simulink model "Dynamics"  (R2023a)
settings: Solver=FixedStepAuto  StartTime=0.0  StopTime=inf  FixedStep=0.001  EnableMultiTasking=on
libraries: sharedutil x32, sharedtransform x18, dspmtrx3 x12, matrix_library x6, simulink_extras x1, simulink x1
(part 3 of 6)

== system Dynamics/Subsystem/M(q),C(q,dq),g(q)/G gen ==
  m : Inport
  Demux : Demux  Outputs=6
  Mux : Mux  Inputs=7
  Product{,1..5} (6 alike) : Product
  g : Constant  Value=[0;0;9.81]
  g1 : Constant  Value=zeros(18,1)
  G : Outport
  wires:
  m/1 -> Demux/1
  Demux/1 -> Product/1
  Demux/2 -> Product1/1
  Demux/3 -> Product2/1
  g/1 -> Product5/2, Product4/2, Product3/2, Product2/2, Product1/2, Product/2
  Demux/4 -> Product3/1
  Demux/5 -> Product4/1
  Demux/6 -> Product5/1
  Product1/1 -> Mux/2
  Product/1 -> Mux/1
  Product2/1 -> Mux/3
  Product4/1 -> Mux/5
  Product5/1 -> Mux/6
  Product3/1 -> Mux/4
  g1/1 -> Mux/7
  Mux/1 -> G/1

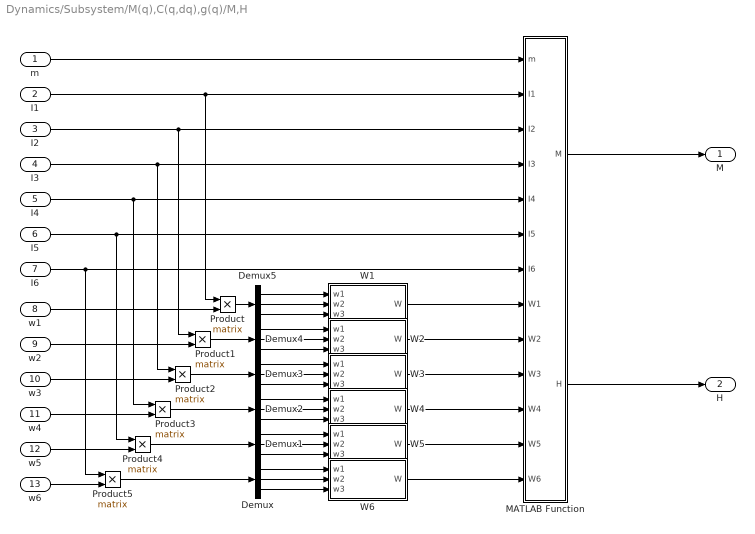
== system Dynamics/Subsystem/M(q),C(q,dq),g(q)/M,H ==
  m : Inport
  I1 : Inport  Port=2
  I2 : Inport  Port=3
  I3 : Inport  Port=4
  I4 : Inport  Port=5
  I5 : Inport  Port=6
  I6 : Inport  Port=7
  w1 : Inport  Port=8
  w2 : Inport  Port=9
  w3 : Inport  Port=10
  w4 : Inport  Port=11
  w5 : Inport  Port=12
  w6 : Inport  Port=13
  Demux{,1..5} (6 alike) : Demux  Outputs=3
  MATLAB Function : MATLAB Function  TreatAsAtomicUnit=on
  Product{,1..5} (6 alike) : Product  Multiplication=Matrix(*)
  W1 : MATLAB Function  TreatAsAtomicUnit=on
  W2 : MATLAB Function  TreatAsAtomicUnit=on
  W3 : MATLAB Function  TreatAsAtomicUnit=on
  W4 : MATLAB Function  TreatAsAtomicUnit=on
  W5 : MATLAB Function  TreatAsAtomicUnit=on
  W6 : MATLAB Function  TreatAsAtomicUnit=on
  M : Outport
  H : Outport  Port=2
  wires:
  m/1 -> MATLAB Function/1(m)
  I1/1 -> Product/1, MATLAB Function/2(I1)
  I2/1 -> Product1/1, MATLAB Function/3(I2)
  I3/1 -> Product2/1, MATLAB Function/4(I3)
  I4/1 -> Product3/1, MATLAB Function/5(I4)
  I5/1 -> Product4/1, MATLAB Function/6(I5)
  I6/1 -> Product5/1, MATLAB Function/7(I6)
  MATLAB Function/1(M) -> M/1
  MATLAB Function/2(H) -> H/1
  W1/1(W) -> MATLAB Function/8(W1)
  W2/1(W) -> MATLAB Function/9(W2)
  W3/1(W) -> MATLAB Function/10(W3)
  W4/1(W) -> MATLAB Function/11(W4)
  W5/1(W) -> MATLAB Function/12(W5)
  W6/1(W) -> MATLAB Function/13(W6)
  w6/1 -> Product5/2
  Demux/3 -> W6/3(w3)
  Demux/2 -> W6/2(w2)
  Demux/1 -> W6/1(w1)
  w5/1 -> Product4/2
  Demux1/3 -> W5/3(w3)
  Demux1/2 -> W5/2(w2)
  Demux1/1 -> W5/1(w1)
  w4/1 -> Product3/2
  Demux2/3 -> W4/3(w3)
  Demux2/2 -> W4/2(w2)
  Demux2/1 -> W4/1(w1)
  w3/1 -> Product2/2
  Demux3/3 -> W3/3(w3)
  Demux3/2 -> W3/2(w2)
  Demux3/1 -> W3/1(w1)
  w2/1 -> Product1/2
  Demux4/3 -> W2/3(w3)
  Demux4/2 -> W2/2(w2)
  Demux4/1 -> W2/1(w1)
  w1/1 -> Product/2
  Demux5/3 -> W1/3(w3)
  Demux5/2 -> W1/2(w2)
  Demux5/1 -> W1/1(w1)
  Product/1 -> Demux5/1
  Product1/1 -> Demux4/1
  Product2/1 -> Demux3/1
  Product3/1 -> Demux2/1
  Product4/1 -> Demux1/1
  Product5/1 -> Demux/1

== system Dynamics/Subsystem/Moments of inertia/Ix, Iy ==
  r : Inport
  m : Inport  Port=2
  h : Inport  Port=3
  Add : Sum
  Gain : Gain  Gain=3
  Gain1 : Gain  Gain=1/12
  Product : Product
  Product1 : Product
  Product2 : Product
  Iz : Outport
  wires:
  r/1 -> Product/1, Product/2
  h/1 -> Product1/1, Product1/2
  Product/1 -> Gain/1
  Product1/1 -> Add/2
  Add/1 -> Product2/1
  m/1 -> Product2/2
  Gain/1 -> Add/1
  Product2/1 -> Gain1/1
  Gain1/1 -> Iz/1

== system Dynamics/Subsystem/Moments of inertia/Ix, Iy1 ==
  r : Inport
  m : Inport  Port=2
  h : Inport  Port=3
  Add : Sum
  Gain : Gain  Gain=3
  Gain1 : Gain  Gain=1/12
  Product : Product
  Product1 : Product
  Product2 : Product
  Iz : Outport
  wires:
  r/1 -> Product/1, Product/2
  h/1 -> Product1/1, Product1/2
  Product/1 -> Gain/1
  Product1/1 -> Add/2
  Add/1 -> Product2/1
  m/1 -> Product2/2
  Gain/1 -> Add/1
  Product2/1 -> Gain1/1
  Gain1/1 -> Iz/1

== system Dynamics/Subsystem/Moments of inertia/Ix, Iy2 ==
  r : Inport
  m : Inport  Port=2
  h : Inport  Port=3
  Add : Sum
  Gain : Gain  Gain=3
  Gain1 : Gain  Gain=1/12
  Product : Product
  Product1 : Product
  Product2 : Product
  Iz : Outport
  wires:
  r/1 -> Product/1, Product/2
  h/1 -> Product1/1, Product1/2
  Product/1 -> Gain/1
  Product1/1 -> Add/2
  Add/1 -> Product2/1
  m/1 -> Product2/2
  Gain/1 -> Add/1
  Product2/1 -> Gain1/1
  Gain1/1 -> Iz/1

== system Dynamics/Subsystem/Moments of inertia/Ix, Iy3 ==
  r : Inport
  m : Inport  Port=2
  h : Inport  Port=3
  Add : Sum
  Gain : Gain  Gain=3
  Gain1 : Gain  Gain=1/12
  Product : Product
  Product1 : Product
  Product2 : Product
  Iz : Outport
  wires:
  r/1 -> Product/1, Product/2
  h/1 -> Product1/1, Product1/2
  Product/1 -> Gain/1
  Product1/1 -> Add/2
  Add/1 -> Product2/1
  m/1 -> Product2/2
  Gain/1 -> Add/1
  Product2/1 -> Gain1/1
  Gain1/1 -> Iz/1

== system Dynamics/Subsystem/Moments of inertia/Ix, Iy4 ==
  r : Inport
  m : Inport  Port=2
  h : Inport  Port=3
  Add : Sum
  Gain : Gain  Gain=3
  Gain1 : Gain  Gain=1/12
  Product : Product
  Product1 : Product
  Product2 : Product
  Iz : Outport
  wires:
  r/1 -> Product/1, Product/2
  h/1 -> Product1/1, Product1/2
  Product/1 -> Gain/1
  Product1/1 -> Add/2
  Add/1 -> Product2/1
  m/1 -> Product2/2
  Gain/1 -> Add/1
  Product2/1 -> Gain1/1
  Gain1/1 -> Iz/1

== system Dynamics/Subsystem/Moments of inertia/Ix, Iy5 ==
  r : Inport
  m : Inport  Port=2
  h : Inport  Port=3
  Add : Sum
  Gain : Gain  Gain=3
  Gain1 : Gain  Gain=1/12
  Product : Product
  Product1 : Product
  Product2 : Product
  Iz : Outport
  wires:
  r/1 -> Product/1, Product/2
  h/1 -> Product1/1, Product1/2
  Product/1 -> Gain/1
  Product1/1 -> Add/2
  Add/1 -> Product2/1
  m/1 -> Product2/2
  Gain/1 -> Add/1
  Product2/1 -> Gain1/1
  Gain1/1 -> Iz/1

== system Dynamics/Subsystem/Moments of inertia/Iz ==
  r : Inport
  m : Inport  Port=2
  Constant : Constant  Value=0.5
  Product : Product  Inputs=4
  Iz : Outport
  wires:
  m/1 -> Product/3
  Constant/1 -> Product/4
  r/1 -> Product/2, Product/1
  Product/1 -> Iz/1

== system Dynamics/Subsystem/Moments of inertia/Iz1 ==
  r : Inport
  m : Inport  Port=2
  Constant : Constant  Value=0.5
  Product : Product  Inputs=4
  Iz : Outport
  wires:
  m/1 -> Product/3
  Constant/1 -> Product/4
  r/1 -> Product/2, Product/1
  Product/1 -> Iz/1

== system Dynamics/Subsystem/Moments of inertia/Iz2 ==
  r : Inport
  m : Inport  Port=2
  Constant : Constant  Value=0.5
  Product : Product  Inputs=4
  Iz : Outport
  wires:
  m/1 -> Product/3
  Constant/1 -> Product/4
  r/1 -> Product/2, Product/1
  Product/1 -> Iz/1

== system Dynamics/Subsystem/Moments of inertia/Iz3 ==
  r : Inport
  m : Inport  Port=2
  Constant : Constant  Value=0.5
  Product : Product  Inputs=4
  Iz : Outport
  wires:
  m/1 -> Product/3
  Constant/1 -> Product/4
  r/1 -> Product/2, Product/1
  Product/1 -> Iz/1

== system Dynamics/Subsystem/Moments of inertia/Iz4 ==
  r : Inport
  m : Inport  Port=2
  Constant : Constant  Value=0.5
  Product : Product  Inputs=4
  Iz : Outport
  wires:
  m/1 -> Product/3
  Constant/1 -> Product/4
  r/1 -> Product/2, Product/1
  Product/1 -> Iz/1

== system Dynamics/Subsystem/Moments of inertia/Iz5 ==
  r : Inport
  m : Inport  Port=2
  Constant : Constant  Value=0.5
  Product : Product  Inputs=4
  Iz : Outport
  wires:
  m/1 -> Product/3
  Constant/1 -> Product/4
  r/1 -> Product/2, Product/1
  Product/1 -> Iz/1

== system Dynamics/Subsystem/Slotine/S-gen ==
  dq : Inport
  V : Inport  Port=2
  Gain : Gain  Gain=-1
  Sum : Sum  Inputs=|++
  S : Outport
  wires:
  dq/1 -> Sum/1
  Sum/1 -> S/1
  V/1 -> Gain/1
  Gain/1 -> Sum/2

== system Dynamics/Subsystem/Slotine/V-gen ==
  q_tilde : Inport
  dq_d : Inport  Port=2
  Gamma : Inport  Port=3
  Gain : Gain  Gain=-1
  Product : Product  Multiplication=Matrix(*)
  Sum : Sum  Inputs=|++
  V : Outport
  wires:
  Gamma/1 -> Product/1
  q_tilde/1 -> Product/2
  Product/1 -> Gain/1
  Sum/1 -> V/1
  dq_d/1 -> Sum/1
  Gain/1 -> Sum/2

== system Dynamics/Subsystem/Slotine/dV-gen ==
  dq_tilde : Inport
  ddq_d : Inport  Port=2
  Gamma : Inport  Port=3
  Gain : Gain  Gain=-1
  Product : Product  Multiplication=Matrix(*)
  Sum : Sum  Inputs=|++
  dV : Outport
  wires:
  Gamma/1 -> Product/1
  dq_tilde/1 -> Product/2
  Product/1 -> Gain/1
  Sum/1 -> dV/1
  ddq_d/1 -> Sum/1
  Gain/1 -> Sum/2

== system Dynamics/Subsystem/Slotine/tau-gen ==
  M : Inport
  C : Inport  Port=2
  g : Inport  Port=3
  V : Inport  Port=4
  dV : Inport  Port=5
  S : Inport  Port=6
  K : Inport  Port=7
  u0 : Inport  Port=8
  Product : Product  Multiplication=Matrix(*)
  Product1 : Product  Multiplication=Matrix(*)
  Product2 : Product  Multiplication=Matrix(*)
  Sum : Sum  Inputs=|++
  Sum1 : Sum  Inputs=|++
  Sum2 : Sum  Inputs=|+-
  Sum3 : Sum  Inputs=|++
  tau : Outport
  wires:
  M/1 -> Product/1
  dV/1 -> Product/2
  C/1 -> Product1/1
  V/1 -> Product1/2
  S/1 -> Product2/2
  K/1 -> Product2/1
  Product/1 -> Sum/1
  Product1/1 -> Sum/2
  Sum/1 -> Sum1/1
  g/1 -> Sum1/2
  Product2/1 -> Sum2/2
  Sum1/1 -> Sum2/1
  Sum2/1 -> Sum3/1
  Sum3/1 -> tau/1
  u0/1 -> Sum3/2

== system Dynamics/Subsystem/Slotine/u0-gen ==
  S : Inport
  sigma(t) : Inport  Port=2
  Divide : Product  Inputs=*/
  Dot Product : DotProduct  OutDataTypeStr=Inherit: Inherit via internal rule
  Gain : Gain  Gain=-1
  Product : Product
  Product1 : Product
  Product2 : Product
  Sqrt : Sqrt
  Sum : Sum  Inputs=|++
  gamma_hat : Integrator  InitialCondition=1
  u0 : Outport
  wires:
  gamma_hat/1 -> Product2/1, Product/2, Product/1
  Dot Product/1 -> Sqrt/1
  S/1 -> Product1/2, Dot Product/2, Dot Product/1
  Sqrt/1 -> Product2/2, gamma_hat/1
  Product/1 -> Product1/1
  Product1/1 -> Divide/1
  Product2/1 -> Sum/1
  Sum/1 -> Divide/2
  sigma(t)/1 -> Sum/2
  Divide/1 -> Gain/1
  Gain/1 -> u0/1

== system Dynamics/Subsystem2/H_6^0/H_1^0 ==
  a : Inport
  alpha : Inport  Port=2
  theta : Inport  Port=3
  d : Inport  Port=4
  Gain1 : Gain  Gain=-1
  Gain2 : Gain  Gain=-1
  MATLAB Function : MATLAB Function  TreatAsAtomicUnit=on
  Mux : Mux  Inputs=3
  Mux1 : Mux  Inputs=3
  Product : Product
  Product1 : Product
  Rotation Angles to Direction Cosine Matrix : sharedtransform/Rotation Angles to Direction Cosine Matrix  rotationOrder=ZXY  aMode=aMode
  Trigonometric Function : Trigonometry  Operator=cos
  Trigonometric Function1 : Trigonometry
  Zero : Constant  Value=0
  H : Outport
  R : Outport  Port=2
  p : Outport  Port=3
  wires:
  Mux/1 -> Rotation Angles to Direction Cosine Matrix/1
  alpha/1 -> Gain1/1
  Zero/1 -> Mux/3
  Rotation Angles to Direction Cosine Matrix/1 -> MATLAB Function/1(R), R/1
  Mux1/1 -> MATLAB Function/2(p), p/1
  Trigonometric Function/1 -> Product/1
  Trigonometric Function1/1 -> Product1/1
  Product/1 -> Mux1/1
  Product1/1 -> Mux1/2
  a/1 -> Product/2, Product1/2
  MATLAB Function/1(H) -> H/1
  Gain1/1 -> Mux/1
  Gain2/1 -> Mux/2
  theta/1 -> Trigonometric Function1/1, Trigonometric Function/1, Gain2/1
  d/1 -> Mux1/3

== system Dynamics/Subsystem2/H_6^0/H_2^1 ==
  a : Inport
  alpha : Inport  Port=2
  theta : Inport  Port=3
  d : Inport  Port=4
  Gain1 : Gain  Gain=-1
  Gain2 : Gain  Gain=-1
  MATLAB Function : MATLAB Function  TreatAsAtomicUnit=on
  Mux : Mux  Inputs=3
  Mux1 : Mux  Inputs=3
  Product : Product
  Product1 : Product
  Rotation Angles to Direction Cosine Matrix : sharedtransform/Rotation Angles to Direction Cosine Matrix  rotationOrder=ZXY  aMode=aMode
  Trigonometric Function : Trigonometry  Operator=cos
  Trigonometric Function1 : Trigonometry
  Zero : Constant  Value=0
  H : Outport
  R : Outport  Port=2
  p : Outport  Port=3
  wires:
  Mux/1 -> Rotation Angles to Direction Cosine Matrix/1
  alpha/1 -> Gain1/1
  Zero/1 -> Mux/3
  Rotation Angles to Direction Cosine Matrix/1 -> MATLAB Function/1(R), R/1
  Mux1/1 -> MATLAB Function/2(p), p/1
  Trigonometric Function/1 -> Product/1
  Trigonometric Function1/1 -> Product1/1
  Product/1 -> Mux1/1
  Product1/1 -> Mux1/2
  a/1 -> Product/2, Product1/2
  MATLAB Function/1(H) -> H/1
  Gain1/1 -> Mux/1
  Gain2/1 -> Mux/2
  theta/1 -> Trigonometric Function1/1, Trigonometric Function/1, Gain2/1
  d/1 -> Mux1/3

== system Dynamics/Subsystem2/H_6^0/H_3^2 ==
  a : Inport
  alpha : Inport  Port=2
  theta : Inport  Port=3
  d : Inport  Port=4
  Gain1 : Gain  Gain=-1
  Gain2 : Gain  Gain=-1
  MATLAB Function : MATLAB Function  TreatAsAtomicUnit=on
  Mux : Mux  Inputs=3
  Mux1 : Mux  Inputs=3
  Product : Product
  Product1 : Product
  Rotation Angles to Direction Cosine Matrix : sharedtransform/Rotation Angles to Direction Cosine Matrix  rotationOrder=ZXY  aMode=aMode
  Trigonometric Function : Trigonometry  Operator=cos
  Trigonometric Function1 : Trigonometry
  Zero : Constant  Value=0
  H : Outport
  R : Outport  Port=2
  p : Outport  Port=3
  wires:
  Mux/1 -> Rotation Angles to Direction Cosine Matrix/1
  alpha/1 -> Gain1/1
  Zero/1 -> Mux/3
  Rotation Angles to Direction Cosine Matrix/1 -> MATLAB Function/1(R), R/1
  Mux1/1 -> MATLAB Function/2(p), p/1
  Trigonometric Function/1 -> Product/1
  Trigonometric Function1/1 -> Product1/1
  Product/1 -> Mux1/1
  Product1/1 -> Mux1/2
  a/1 -> Product/2, Product1/2
  MATLAB Function/1(H) -> H/1
  Gain1/1 -> Mux/1
  Gain2/1 -> Mux/2
  theta/1 -> Trigonometric Function1/1, Trigonometric Function/1, Gain2/1
  d/1 -> Mux1/3

== system Dynamics/Subsystem2/H_6^0/H_4^3 ==
  a : Inport
  alpha : Inport  Port=2
  theta : Inport  Port=3
  d : Inport  Port=4
  Gain1 : Gain  Gain=-1
  Gain2 : Gain  Gain=-1
  MATLAB Function : MATLAB Function  TreatAsAtomicUnit=on
  Mux : Mux  Inputs=3
  Mux1 : Mux  Inputs=3
  Product : Product
  Product1 : Product
  Rotation Angles to Direction Cosine Matrix : sharedtransform/Rotation Angles to Direction Cosine Matrix  rotationOrder=ZXY  aMode=aMode
  Trigonometric Function : Trigonometry  Operator=cos
  Trigonometric Function1 : Trigonometry
  Zero : Constant  Value=0
  H : Outport
  R : Outport  Port=2
  p : Outport  Port=3
  wires:
  Mux/1 -> Rotation Angles to Direction Cosine Matrix/1
  alpha/1 -> Gain1/1
  Zero/1 -> Mux/3
  Rotation Angles to Direction Cosine Matrix/1 -> MATLAB Function/1(R), R/1
  Mux1/1 -> MATLAB Function/2(p), p/1
  Trigonometric Function/1 -> Product/1
  Trigonometric Function1/1 -> Product1/1
  Product/1 -> Mux1/1
  Product1/1 -> Mux1/2
  a/1 -> Product/2, Product1/2
  MATLAB Function/1(H) -> H/1
  Gain1/1 -> Mux/1
  Gain2/1 -> Mux/2
  theta/1 -> Trigonometric Function1/1, Trigonometric Function/1, Gain2/1
  d/1 -> Mux1/3

== system Dynamics/Subsystem2/H_6^0/H_5^4 ==
  a : Inport
  alpha : Inport  Port=2
  theta : Inport  Port=3
  d : Inport  Port=4
  Gain1 : Gain  Gain=-1
  Gain2 : Gain  Gain=-1
  MATLAB Function : MATLAB Function  TreatAsAtomicUnit=on
  Mux : Mux  Inputs=3
  Mux1 : Mux  Inputs=3
  Product : Product
  Product1 : Product
  Rotation Angles to Direction Cosine Matrix : sharedtransform/Rotation Angles to Direction Cosine Matrix  rotationOrder=ZXY  aMode=aMode
  Trigonometric Function : Trigonometry  Operator=cos
  Trigonometric Function1 : Trigonometry
  Zero : Constant  Value=0
  H : Outport
  R : Outport  Port=2
  p : Outport  Port=3
  wires:
  Mux/1 -> Rotation Angles to Direction Cosine Matrix/1
  alpha/1 -> Gain1/1
  Zero/1 -> Mux/3
  Rotation Angles to Direction Cosine Matrix/1 -> MATLAB Function/1(R), R/1
  Mux1/1 -> MATLAB Function/2(p), p/1
  Trigonometric Function/1 -> Product/1
  Trigonometric Function1/1 -> Product1/1
  Product/1 -> Mux1/1
  Product1/1 -> Mux1/2
  a/1 -> Product/2, Product1/2
  MATLAB Function/1(H) -> H/1
  Gain1/1 -> Mux/1
  Gain2/1 -> Mux/2
  theta/1 -> Trigonometric Function1/1, Trigonometric Function/1, Gain2/1
  d/1 -> Mux1/3

== system Dynamics/Subsystem2/H_6^0/H_6^5 ==
  a : Inport
  alpha : Inport  Port=2
  theta : Inport  Port=3
  d : Inport  Port=4
  Gain1 : Gain  Gain=-1
  Gain2 : Gain  Gain=-1
  MATLAB Function : MATLAB Function  TreatAsAtomicUnit=on
  Mux : Mux  Inputs=3
  Mux1 : Mux  Inputs=3
  Product : Product
  Product1 : Product
  Rotation Angles to Direction Cosine Matrix : sharedtransform/Rotation Angles to Direction Cosine Matrix  rotationOrder=ZXY  aMode=aMode
  Trigonometric Function : Trigonometry  Operator=cos
  Trigonometric Function1 : Trigonometry
  Zero : Constant  Value=0
  H : Outport
  R : Outport  Port=2
  p : Outport  Port=3
  wires:
  Mux/1 -> Rotation Angles to Direction Cosine Matrix/1
  alpha/1 -> Gain1/1
  Zero/1 -> Mux/3
  Rotation Angles to Direction Cosine Matrix/1 -> MATLAB Function/1(R), R/1
  Mux1/1 -> MATLAB Function/2(p), p/1
  Trigonometric Function/1 -> Product/1
  Trigonometric Function1/1 -> Product1/1
  Product/1 -> Mux1/1
  Product1/1 -> Mux1/2
  a/1 -> Product/2, Product1/2
  MATLAB Function/1(H) -> H/1
  Gain1/1 -> Mux/1
  Gain2/1 -> Mux/2
  theta/1 -> Trigonometric Function1/1, Trigonometric Function/1, Gain2/1
  d/1 -> Mux1/3

== system Dynamics/Subsystem2/Jacobian/J(q) gen. ==
  R_1^0 : Inport
  R_2^0 : Inport  Port=2
  R_3^0 : Inport  Port=3
  R_4^0 : Inport  Port=4
  R_5^0 : Inport  Port=5
  R_6^0 : Inport  Port=6
  p_1^0 : Inport  Port=7
  p_2^0 : Inport  Port=8
  p_3^0 : Inport  Port=9
  p_4^0 : Inport  Port=10
  p_5^0 : Inport  Port=11
  type1 : Inport  Port=12
  type2 : Inport  Port=13
  type3 : Inport  Port=14
  type4 : Inport  Port=15
  J_v_6(q) : Inport  Port=16
  J_w1 : Inport  Port=17
  J_w2 : Inport  Port=18
  J_w3 : Inport  Port=19
  J_w4 : Inport  Port=20
  J_w5 : Inport  Port=21
  J_w6 : Inport  Port=22
  J_v_1(q) : Subsystem
  J_v_2(q) : Subsystem
  J_v_3(q) : Subsystem
  J_v_4(q) : Subsystem
  J_v_5(q) : Subsystem
  MATLAB Function : MATLAB Function  TreatAsAtomicUnit=on
  J(q) : Outport
  wires:
  MATLAB Function/1(J_q) -> J(q)/1
  J_v_6(q)/1 -> MATLAB Function/12(J_v6)
  J_w1/1 -> MATLAB Function/1(J_w1)
  J_w2/1 -> MATLAB Function/2(J_w2)
  J_w3/1 -> MATLAB Function/3(J_w3)
  J_w4/1 -> MATLAB Function/4(J_w4)
  J_w5/1 -> MATLAB Function/5(J_w5)
  J_w6/1 -> MATLAB Function/6(J_w6)
  J_v_1(q)/1(J_v_1(q)) -> MATLAB Function/7(J_v1)
  J_v_2(q)/1(J_v_2(q)) -> MATLAB Function/8(J_v2)
  J_v_3(q)/1(J_v_3(q)) -> MATLAB Function/9(J_v3)
  J_v_4(q)/1(J_v_4(q)) -> MATLAB Function/10(J_v4)
  J_v_5(q)/1(J_v_5(q)) -> MATLAB Function/11(J_v5)
  R_5^0/1 -> MATLAB Function/17(R5)
  R_6^0/1 -> MATLAB Function/18(R6)
  R_1^0/1 -> MATLAB Function/13(R1), J_v_5(q)/1(R_1^0), J_v_4(q)/1(R_1^0), J_v_3(q)/1(R_1^0), J_v_2(q)/1(R_1^0)
  R_2^0/1 -> MATLAB Function/14(R2), J_v_5(q)/2(R_2^0), J_v_4(q)/2(R_2^0), J_v_3(q)/2(R_2^0)
  R_3^0/1 -> J_v_4(q)/3(R_3^0), MATLAB Function/15(R3), J_v_5(q)/3(R_3^0)
  R_4^0/1 -> MATLAB Function/16(R4), J_v_5(q)/4(R_4^0)
  p_1^0/1 -> J_v_5(q)/5(p_1^0), J_v_4(q)/4(p_1^0), J_v_3(q)/3(p_1^0), J_v_2(q)/2(p_1^0)
  p_2^0/1 -> J_v_5(q)/6(p_2^0), J_v_4(q)/5(p_2^0), J_v_3(q)/4(p_2^0), J_v_2(q)/3(p_2^0)
  p_3^0/1 -> J_v_3(q)/5(p_3^0), J_v_5(q)/7(p_3^0), J_v_4(q)/6(p_3^0)
  p_4^0/1 -> J_v_5(q)/8(p_4^0), J_v_4(q)/7(p_4^0)
  p_5^0/1 -> J_v_5(q)/9(p_5^0)
  type1/1 -> J_v_5(q)/10(type1), J_v_4(q)/8(type1), J_v_3(q)/6(type1), J_v_2(q)/4(type1)
  type2/1 -> J_v_5(q)/11(type2), J_v_4(q)/9(type2), J_v_3(q)/7(type2)
  type3/1 -> J_v_5(q)/12(type3), J_v_4(q)/10(type3)
  type4/1 -> J_v_5(q)/13(type4)

== system Dynamics/Subsystem2/Jacobian/J_v ==
  R_1^0 : Inport
  R_2^0 : Inport  Port=2
  R_3^0 : Inport  Port=3
  R_4^0 : Inport  Port=4
  R_5^0 : Inport  Port=5
  R_6^0 : Inport  Port=6
  p_1^0 : Inport  Port=7
  p_2^0 : Inport  Port=8
  p_3^0 : Inport  Port=9
  p_4^0 : Inport  Port=10
  p_5^0 : Inport  Port=11
  p_6^0 : Inport  Port=12
  type1 : Inport  Port=13
  type2 : Inport  Port=14
  type3 : Inport  Port=15
  type4 : Inport  Port=16
  type5 : Inport  Port=17
  type6 : Inport  Port=18
  J_v_1 : Subsystem
  J_v_2 : Subsystem
  J_v_3 : Subsystem
  J_v_4 : Subsystem
  J_v_5 : Subsystem
  J_v_6 : Subsystem
  v2M_1 : MATLAB Function  TreatAsAtomicUnit=on
  v2M_2 : MATLAB Function  TreatAsAtomicUnit=on
  v2M_3 : MATLAB Function  TreatAsAtomicUnit=on
  v2M_4 : MATLAB Function  TreatAsAtomicUnit=on
  v2M_5 : MATLAB Function  TreatAsAtomicUnit=on
  J_v : Outport
  wires:
  R_1^0/1 -> J_v_1/1(R)
  J_v_1/1(J_v) -> v2M_1/1(v1)
  v2M_1/1(M) -> v2M_2/1(v1)
  v2M_2/1(M) -> v2M_3/1(v1)
  v2M_3/1(M) -> v2M_4/1(v1)
  v2M_4/1(M) -> v2M_5/1(v1)
  v2M_5/1(M) -> J_v/1
  J_v_2/1(J_v) -> v2M_1/2(v2)
  J_v_3/1(J_v) -> v2M_2/2(v2)
  J_v_4/1(J_v) -> v2M_3/2(v2)
  J_v_5/1(J_v) -> v2M_4/2(v2)
  J_v_6/1(J_v) -> v2M_5/2(v2)
  R_2^0/1 -> J_v_2/1(R)
  R_3^0/1 -> J_v_3/1(R)
  R_4^0/1 -> J_v_4/1(R)
  R_5^0/1 -> J_v_5/1(R)
  R_6^0/1 -> J_v_6/1(R)
  p_1^0/1 -> J_v_1/2(p)
  p_2^0/1 -> J_v_2/2(p)
  p_3^0/1 -> J_v_3/2(p)
  p_4^0/1 -> J_v_4/2(p)
  p_5^0/1 -> J_v_5/2(p)
  type2/1 -> J_v_2/4(type)
  type1/1 -> J_v_1/4(type)
  type3/1 -> J_v_3/4(type)
  type4/1 -> J_v_4/4(type)
  type5/1 -> J_v_5/4(type)
  type6/1 -> J_v_6/4(type)
  p_6^0/1 -> J_v_6/2(p), J_v_1/3(pn), J_v_2/3(pn), J_v_3/3(pn), J_v_4/3(pn), J_v_5/3(pn), J_v_6/3(pn)

== system Dynamics/Subsystem2/Jacobian/J_w ==
  R_1^0 : Inport
  R_2^0 : Inport  Port=2
  R_3^0 : Inport  Port=3
  R_4^0 : Inport  Port=4
  R_5^0 : Inport  Port=5
  R_6^0 : Inport  Port=6
  type1 : Inport  Port=7
  type2 : Inport  Port=8
  type3 : Inport  Port=9
  type4 : Inport  Port=10
  type5 : Inport  Port=11
  type6 : Inport  Port=12
  J_w_1 : MATLAB Function  TreatAsAtomicUnit=on
  J_w_2 : MATLAB Function  TreatAsAtomicUnit=on
  J_w_3 : MATLAB Function  TreatAsAtomicUnit=on
  J_w_4 : MATLAB Function  TreatAsAtomicUnit=on
  J_w_5 : MATLAB Function  TreatAsAtomicUnit=on
  J_w_6 : MATLAB Function  TreatAsAtomicUnit=on
  v2M_1 : MATLAB Function  TreatAsAtomicUnit=on
  v2M_2 : MATLAB Function  TreatAsAtomicUnit=on
  v2M_3 : MATLAB Function  TreatAsAtomicUnit=on
  v2M_4 : MATLAB Function  TreatAsAtomicUnit=on
  v2M_5 : MATLAB Function  TreatAsAtomicUnit=on
  EF J_w : Outport
  J_w1 : Outport  Port=2
  J_w2 : Outport  Port=3
  J_w3 : Outport  Port=4
  J_w4 : Outport  Port=5
  J_w5 : Outport  Port=6
  J_w6 : Outport  Port=7
  wires:
  R_1^0/1 -> J_w_1/1(R)
  R_2^0/1 -> J_w_2/1(R)
  R_3^0/1 -> J_w_3/1(R)
  R_4^0/1 -> J_w_4/1(R)
  R_5^0/1 -> J_w_5/1(R)
  R_6^0/1 -> J_w_6/1(R)
  J_w_1/1(J_w) -> J_w1/1, v2M_1/1(v1)
  J_w_2/1(J_w) -> J_w2/1, v2M_1/2(v2)
  J_w_3/1(J_w) -> J_w3/1, v2M_2/2(v2)
  v2M_1/1(M) -> v2M_2/1(v1)
  v2M_2/1(M) -> v2M_3/1(v1)
  v2M_3/1(M) -> v2M_4/1(v1)
  J_w_5/1(J_w) -> J_w5/1, v2M_4/2(v2)
  J_w_6/1(J_w) -> J_w6/1, v2M_5/2(v2)
  v2M_4/1(M) -> v2M_5/1(v1)
  v2M_5/1(M) -> EF J_w/1
  type1/1 -> J_w_1/2(type)
  type2/1 -> J_w_2/2(type)
  type3/1 -> J_w_3/2(type)
  type4/1 -> J_w_4/2(type)
  type5/1 -> J_w_5/2(type)
  type6/1 -> J_w_6/2(type)
  J_w_4/1(J_w) -> v2M_3/2(v2), J_w4/1

== system Dynamics/Subsystem2/M(q),C(q,dq),g(q)/G gen ==
  m : Inport
  Demux : Demux  Outputs=6
  Mux : Mux  Inputs=7
  Product{,1..5} (6 alike) : Product
  g : Constant  Value=[0;0;9.81]
  g1 : Constant  Value=zeros(18,1)
  G : Outport
  wires:
  m/1 -> Demux/1
  Demux/1 -> Product/1
  Demux/2 -> Product1/1
  Demux/3 -> Product2/1
  g/1 -> Product5/2, Product4/2, Product3/2, Product2/2, Product1/2, Product/2
  Demux/4 -> Product3/1
  Demux/5 -> Product4/1
  Demux/6 -> Product5/1
  Product1/1 -> Mux/2
  Product/1 -> Mux/1
  Product2/1 -> Mux/3
  Product4/1 -> Mux/5
  Product5/1 -> Mux/6
  Product3/1 -> Mux/4
  g1/1 -> Mux/7
  Mux/1 -> G/1

== system Dynamics/Subsystem2/M(q),C(q,dq),g(q)/M,H ==
  m : Inport
  I1 : Inport  Port=2
  I2 : Inport  Port=3
  I3 : Inport  Port=4
  I4 : Inport  Port=5
  I5 : Inport  Port=6
  I6 : Inport  Port=7
  w1 : Inport  Port=8
  w2 : Inport  Port=9
  w3 : Inport  Port=10
  w4 : Inport  Port=11
  w5 : Inport  Port=12
  w6 : Inport  Port=13
  Demux{,1..5} (6 alike) : Demux  Outputs=3
  MATLAB Function : MATLAB Function  TreatAsAtomicUnit=on
  Product{,1..5} (6 alike) : Product  Multiplication=Matrix(*)
  W1 : MATLAB Function  TreatAsAtomicUnit=on
  W2 : MATLAB Function  TreatAsAtomicUnit=on
  W3 : MATLAB Function  TreatAsAtomicUnit=on
  W4 : MATLAB Function  TreatAsAtomicUnit=on
  W5 : MATLAB Function  TreatAsAtomicUnit=on
  W6 : MATLAB Function  TreatAsAtomicUnit=on
  M : Outport
  H : Outport  Port=2
  wires:
  m/1 -> MATLAB Function/1(m)
  I1/1 -> Product/1, MATLAB Function/2(I1)
  I2/1 -> Product1/1, MATLAB Function/3(I2)
  I3/1 -> Product2/1, MATLAB Function/4(I3)
  I4/1 -> Product3/1, MATLAB Function/5(I4)
  I5/1 -> Product4/1, MATLAB Function/6(I5)
  I6/1 -> Product5/1, MATLAB Function/7(I6)
  MATLAB Function/1(M) -> M/1
  MATLAB Function/2(H) -> H/1
  W1/1(W) -> MATLAB Function/8(W1)
  W2/1(W) -> MATLAB Function/9(W2)
  W3/1(W) -> MATLAB Function/10(W3)
  W4/1(W) -> MATLAB Function/11(W4)
  W5/1(W) -> MATLAB Function/12(W5)
  W6/1(W) -> MATLAB Function/13(W6)
  w6/1 -> Product5/2
  Demux/3 -> W6/3(w3)
  Demux/2 -> W6/2(w2)
  Demux/1 -> W6/1(w1)
  w5/1 -> Product4/2
  Demux1/3 -> W5/3(w3)
  Demux1/2 -> W5/2(w2)
  Demux1/1 -> W5/1(w1)
  w4/1 -> Product3/2
  Demux2/3 -> W4/3(w3)
  Demux2/2 -> W4/2(w2)
  Demux2/1 -> W4/1(w1)
  w3/1 -> Product2/2
  Demux3/3 -> W3/3(w3)
  Demux3/2 -> W3/2(w2)
  Demux3/1 -> W3/1(w1)
  w2/1 -> Product1/2
  Demux4/3 -> W2/3(w3)
  Demux4/2 -> W2/2(w2)
  Demux4/1 -> W2/1(w1)
  w1/1 -> Product/2
  Demux5/3 -> W1/3(w3)
  Demux5/2 -> W1/2(w2)
  Demux5/1 -> W1/1(w1)
  Product/1 -> Demux5/1
  Product1/1 -> Demux4/1
  Product2/1 -> Demux3/1
  Product3/1 -> Demux2/1
  Product4/1 -> Demux1/1
  Product5/1 -> Demux/1

== system Dynamics/Subsystem2/Moments of inertia/Ix, Iy ==
  r : Inport
  m : Inport  Port=2
  h : Inport  Port=3
  Add : Sum
  Gain : Gain  Gain=3
  Gain1 : Gain  Gain=1/12
  Product : Product
  Product1 : Product
  Product2 : Product
  Iz : Outport
  wires:
  r/1 -> Product/1, Product/2
  h/1 -> Product1/1, Product1/2
  Product/1 -> Gain/1
  Product1/1 -> Add/2
  Add/1 -> Product2/1
  m/1 -> Product2/2
  Gain/1 -> Add/1
  Product2/1 -> Gain1/1
  Gain1/1 -> Iz/1

== system Dynamics/Subsystem2/Moments of inertia/Ix, Iy1 ==
  r : Inport
  m : Inport  Port=2
  h : Inport  Port=3
  Add : Sum
  Gain : Gain  Gain=3
  Gain1 : Gain  Gain=1/12
  Product : Product
  Product1 : Product
  Product2 : Product
  Iz : Outport
  wires:
  r/1 -> Product/1, Product/2
  h/1 -> Product1/1, Product1/2
  Product/1 -> Gain/1
  Product1/1 -> Add/2
  Add/1 -> Product2/1
  m/1 -> Product2/2
  Gain/1 -> Add/1
  Product2/1 -> Gain1/1
  Gain1/1 -> Iz/1

== system Dynamics/Subsystem2/Moments of inertia/Ix, Iy2 ==
  r : Inport
  m : Inport  Port=2
  h : Inport  Port=3
  Add : Sum
  Gain : Gain  Gain=3
  Gain1 : Gain  Gain=1/12
  Product : Product
  Product1 : Product
  Product2 : Product
  Iz : Outport
  wires:
  r/1 -> Product/1, Product/2
  h/1 -> Product1/1, Product1/2
  Product/1 -> Gain/1
  Product1/1 -> Add/2
  Add/1 -> Product2/1
  m/1 -> Product2/2
  Gain/1 -> Add/1
  Product2/1 -> Gain1/1
  Gain1/1 -> Iz/1

== system Dynamics/Subsystem2/Moments of inertia/Ix, Iy3 ==
  r : Inport
  m : Inport  Port=2
  h : Inport  Port=3
  Add : Sum
  Gain : Gain  Gain=3
  Gain1 : Gain  Gain=1/12
  Product : Product
  Product1 : Product
  Product2 : Product
  Iz : Outport
  wires:
  r/1 -> Product/1, Product/2
  h/1 -> Product1/1, Product1/2
  Product/1 -> Gain/1
  Product1/1 -> Add/2
  Add/1 -> Product2/1
  m/1 -> Product2/2
  Gain/1 -> Add/1
  Product2/1 -> Gain1/1
  Gain1/1 -> Iz/1

== system Dynamics/Subsystem2/Moments of inertia/Ix, Iy4 ==
  r : Inport
  m : Inport  Port=2
  h : Inport  Port=3
  Add : Sum
  Gain : Gain  Gain=3
  Gain1 : Gain  Gain=1/12
  Product : Product
  Product1 : Product
  Product2 : Product
  Iz : Outport
  wires:
  r/1 -> Product/1, Product/2
  h/1 -> Product1/1, Product1/2
  Product/1 -> Gain/1
  Product1/1 -> Add/2
  Add/1 -> Product2/1
  m/1 -> Product2/2
  Gain/1 -> Add/1
  Product2/1 -> Gain1/1
  Gain1/1 -> Iz/1

== system Dynamics/Subsystem2/Moments of inertia/Ix, Iy5 ==
  r : Inport
  m : Inport  Port=2
  h : Inport  Port=3
  Add : Sum
  Gain : Gain  Gain=3
  Gain1 : Gain  Gain=1/12
  Product : Product
  Product1 : Product
  Product2 : Product
  Iz : Outport
  wires:
  r/1 -> Product/1, Product/2
  h/1 -> Product1/1, Product1/2
  Product/1 -> Gain/1
  Product1/1 -> Add/2
  Add/1 -> Product2/1
  m/1 -> Product2/2
  Gain/1 -> Add/1
  Product2/1 -> Gain1/1
  Gain1/1 -> Iz/1

== system Dynamics/Subsystem2/Moments of inertia/Iz ==
  r : Inport
  m : Inport  Port=2
  Constant : Constant  Value=0.5
  Product : Product  Inputs=4
  Iz : Outport
  wires:
  m/1 -> Product/3
  Constant/1 -> Product/4
  r/1 -> Product/2, Product/1
  Product/1 -> Iz/1

== system Dynamics/Subsystem2/Moments of inertia/Iz1 ==
  r : Inport
  m : Inport  Port=2
  Constant : Constant  Value=0.5
  Product : Product  Inputs=4
  Iz : Outport
  wires:
  m/1 -> Product/3
  Constant/1 -> Product/4
  r/1 -> Product/2, Product/1
  Product/1 -> Iz/1

== system Dynamics/Subsystem2/Moments of inertia/Iz2 ==
  r : Inport
  m : Inport  Port=2
  Constant : Constant  Value=0.5
  Product : Product  Inputs=4
  Iz : Outport
  wires:
  m/1 -> Product/3
  Constant/1 -> Product/4
  r/1 -> Product/2, Product/1
  Product/1 -> Iz/1

== system Dynamics/Subsystem2/Moments of inertia/Iz3 ==
  r : Inport
  m : Inport  Port=2
  Constant : Constant  Value=0.5
  Product : Product  Inputs=4
  Iz : Outport
  wires:
  m/1 -> Product/3
  Constant/1 -> Product/4
  r/1 -> Product/2, Product/1
  Product/1 -> Iz/1

== system Dynamics/Subsystem2/Moments of inertia/Iz4 ==
  r : Inport
  m : Inport  Port=2
  Constant : Constant  Value=0.5
  Product : Product  Inputs=4
  Iz : Outport
  wires:
  m/1 -> Product/3
  Constant/1 -> Product/4
  r/1 -> Product/2, Product/1
  Product/1 -> Iz/1

== system Dynamics/Subsystem2/Moments of inertia/Iz5 ==
  r : Inport
  m : Inport  Port=2
  Constant : Constant  Value=0.5
  Product : Product  Inputs=4
  Iz : Outport
  wires:
  m/1 -> Product/3
  Constant/1 -> Product/4
  r/1 -> Product/2, Product/1
  Product/1 -> Iz/1

== system Dynamics/Subsystem2/Slotine/S-gen ==
  dq : Inport
  V : Inport  Port=2
  Gain : Gain  Gain=-1
  Sum : Sum  Inputs=|++
  S : Outport
  wires:
  dq/1 -> Sum/1
  Sum/1 -> S/1
  V/1 -> Gain/1
  Gain/1 -> Sum/2

== system Dynamics/Subsystem2/Slotine/V-gen ==
  q_tilde : Inport
  dq_d : Inport  Port=2
  Gamma : Inport  Port=3
  Gain : Gain  Gain=-1
  Product : Product  Multiplication=Matrix(*)
  Sum : Sum  Inputs=|++
  V : Outport
  wires:
  Gamma/1 -> Product/1
  q_tilde/1 -> Product/2
  Product/1 -> Gain/1
  Sum/1 -> V/1
  dq_d/1 -> Sum/1
  Gain/1 -> Sum/2

== system Dynamics/Subsystem2/Slotine/dV-gen ==
  dq_tilde : Inport
  ddq_d : Inport  Port=2
  Gamma : Inport  Port=3
  Gain : Gain  Gain=-1
  Product : Product  Multiplication=Matrix(*)
  Sum : Sum  Inputs=|++
  dV : Outport
  wires:
  Gamma/1 -> Product/1
  dq_tilde/1 -> Product/2
  Product/1 -> Gain/1
  Sum/1 -> dV/1
  ddq_d/1 -> Sum/1
  Gain/1 -> Sum/2

== system Dynamics/Subsystem2/Slotine/tau-gen ==
  M : Inport
  C : Inport  Port=2
  g : Inport  Port=3
  V : Inport  Port=4
  dV : Inport  Port=5
  S : Inport  Port=6
  K : Inport  Port=7
  Product : Product  Multiplication=Matrix(*)
  Product1 : Product  Multiplication=Matrix(*)
  Product2 : Product  Multiplication=Matrix(*)
  Sum : Sum  Inputs=|++
  Sum1 : Sum  Inputs=|++
  Sum2 : Sum  Inputs=|+-
  tau : Outport
  wires:
  M/1 -> Product/1
  dV/1 -> Product/2
  C/1 -> Product1/1
  V/1 -> Product1/2
  S/1 -> Product2/2
  K/1 -> Product2/1
  Product/1 -> Sum/1
  Product1/1 -> Sum/2
  Sum/1 -> Sum1/1
  g/1 -> Sum1/2
  Product2/1 -> Sum2/2
  Sum1/1 -> Sum2/1
  Sum2/1 -> tau/1

== system Dynamics/DYNAMIC/Jacobian/J(q) gen./J_v_1(q) ==
  Constant : Constant  Value=zeros(3,1)
  v2M_1 : MATLAB Function  TreatAsAtomicUnit=on
  v2M_2 : MATLAB Function  TreatAsAtomicUnit=on
  v2M_3 : MATLAB Function  TreatAsAtomicUnit=on
  v2M_4 : MATLAB Function  TreatAsAtomicUnit=on
  v2M_5 : MATLAB Function  TreatAsAtomicUnit=on
  J_v_1(q) : Outport
  wires:
  Constant/1 -> v2M_1/1(v1), v2M_5/2(v2), v2M_4/2(v2), v2M_3/2(v2), v2M_2/2(v2), v2M_1/2(v2)
  v2M_1/1(M) -> v2M_2/1(v1)
  v2M_2/1(M) -> v2M_3/1(v1)
  v2M_3/1(M) -> v2M_4/1(v1)
  v2M_4/1(M) -> v2M_5/1(v1)
  v2M_5/1(M) -> J_v_1(q)/1

== system Dynamics/DYNAMIC/Jacobian/J(q) gen./J_v_2(q) ==
  R_1^0 : Inport
  p_1^0 : Inport  Port=2
  p_2^0 : Inport  Port=3
  type1 : Inport  Port=4
  Constant : Constant  Value=zeros(3,1)
  J_v_1 : Subsystem
  v2M_1 : MATLAB Function  TreatAsAtomicUnit=on
  v2M_2 : MATLAB Function  TreatAsAtomicUnit=on
  v2M_3 : MATLAB Function  TreatAsAtomicUnit=on
  v2M_4 : MATLAB Function  TreatAsAtomicUnit=on
  v2M_5 : MATLAB Function  TreatAsAtomicUnit=on
  J_v_2(q) : Outport
  wires:
  R_1^0/1 -> J_v_1/1(R)
  J_v_1/1(J_v) -> v2M_1/1(v1)
  v2M_1/1(M) -> v2M_2/1(v1)
  v2M_2/1(M) -> v2M_3/1(v1)
  v2M_3/1(M) -> v2M_4/1(v1)
  v2M_4/1(M) -> v2M_5/1(v1)
  v2M_5/1(M) -> J_v_2(q)/1
  Constant/1 -> v2M_3/2(v2), v2M_4/2(v2), v2M_5/2(v2), v2M_1/2(v2), v2M_2/2(v2)
  p_1^0/1 -> J_v_1/2(p)
  type1/1 -> J_v_1/4(type)
  p_2^0/1 -> J_v_1/3(pn)

== system Dynamics/DYNAMIC/Jacobian/J(q) gen./J_v_3(q) ==
  R_1^0 : Inport
  R_2^0 : Inport  Port=2
  p_1^0 : Inport  Port=3
  p_2^0 : Inport  Port=4
  p_3^0 : Inport  Port=5
  type1 : Inport  Port=6
  type2 : Inport  Port=7
  Constant : Constant  Value=zeros(3,1)
  J_v_1 : Subsystem
  J_v_2 : Subsystem
  v2M_1 : MATLAB Function  TreatAsAtomicUnit=on
  v2M_2 : MATLAB Function  TreatAsAtomicUnit=on
  v2M_3 : MATLAB Function  TreatAsAtomicUnit=on
  v2M_4 : MATLAB Function  TreatAsAtomicUnit=on
  v2M_5 : MATLAB Function  TreatAsAtomicUnit=on
  J_v_3(q) : Outport
  wires:
  R_1^0/1 -> J_v_1/1(R)
  J_v_1/1(J_v) -> v2M_1/1(v1)
  v2M_1/1(M) -> v2M_2/1(v1)
  v2M_2/1(M) -> v2M_3/1(v1)
  v2M_3/1(M) -> v2M_4/1(v1)
  v2M_4/1(M) -> v2M_5/1(v1)
  v2M_5/1(M) -> J_v_3(q)/1
  J_v_2/1(J_v) -> v2M_1/2(v2)
  Constant/1 -> v2M_5/2(v2), v2M_4/2(v2), v2M_2/2(v2), v2M_3/2(v2)
  R_2^0/1 -> J_v_2/1(R)
  p_1^0/1 -> J_v_1/2(p)
  p_2^0/1 -> J_v_2/2(p)
  type2/1 -> J_v_2/4(type)
  type1/1 -> J_v_1/4(type)
  p_3^0/1 -> J_v_1/3(pn), J_v_2/3(pn)

== system Dynamics/DYNAMIC/Jacobian/J(q) gen./J_v_4(q) ==
  R_1^0 : Inport
  R_2^0 : Inport  Port=2
  R_3^0 : Inport  Port=3
  p_1^0 : Inport  Port=4
  p_2^0 : Inport  Port=5
  p_3^0 : Inport  Port=6
  p_4^0 : Inport  Port=7
  type1 : Inport  Port=8
  type2 : Inport  Port=9
  type3 : Inport  Port=10
  Constant : Constant  Value=zeros(3,1)
  J_v_1 : Subsystem
  J_v_2 : Subsystem
  J_v_3 : Subsystem
  v2M_1 : MATLAB Function  TreatAsAtomicUnit=on
  v2M_2 : MATLAB Function  TreatAsAtomicUnit=on
  v2M_3 : MATLAB Function  TreatAsAtomicUnit=on
  v2M_4 : MATLAB Function  TreatAsAtomicUnit=on
  v2M_5 : MATLAB Function  TreatAsAtomicUnit=on
  J_v_4(q) : Outport
  wires:
  R_1^0/1 -> J_v_1/1(R)
  J_v_1/1(J_v) -> v2M_1/1(v1)
  v2M_1/1(M) -> v2M_2/1(v1)
  v2M_2/1(M) -> v2M_3/1(v1)
  v2M_3/1(M) -> v2M_4/1(v1)
  v2M_4/1(M) -> v2M_5/1(v1)
  v2M_5/1(M) -> J_v_4(q)/1
  J_v_2/1(J_v) -> v2M_1/2(v2)
  J_v_3/1(J_v) -> v2M_2/2(v2)
  Constant/1 -> v2M_5/2(v2), v2M_3/2(v2), v2M_4/2(v2)
  R_2^0/1 -> J_v_2/1(R)
  R_3^0/1 -> J_v_3/1(R)
  p_1^0/1 -> J_v_1/2(p)
  p_2^0/1 -> J_v_2/2(p)
  p_3^0/1 -> J_v_3/2(p)
  type2/1 -> J_v_2/4(type)
  type1/1 -> J_v_1/4(type)
  type3/1 -> J_v_3/4(type)
  p_4^0/1 -> J_v_1/3(pn), J_v_2/3(pn), J_v_3/3(pn)

== system Dynamics/DYNAMIC/Jacobian/J(q) gen./J_v_5(q) ==
  R_1^0 : Inport
  R_2^0 : Inport  Port=2
  R_3^0 : Inport  Port=3
  R_4^0 : Inport  Port=4
  p_1^0 : Inport  Port=5
  p_2^0 : Inport  Port=6
  p_3^0 : Inport  Port=7
  p_4^0 : Inport  Port=8
  p_5^0 : Inport  Port=9
  type1 : Inport  Port=10
  type2 : Inport  Port=11
  type3 : Inport  Port=12
  type4 : Inport  Port=13
  Constant : Constant  Value=zeros(3,1)
  J_v_1 : Subsystem
  J_v_2 : Subsystem
  J_v_3 : Subsystem
  J_v_4 : Subsystem
  v2M_1 : MATLAB Function  TreatAsAtomicUnit=on
  v2M_2 : MATLAB Function  TreatAsAtomicUnit=on
  v2M_3 : MATLAB Function  TreatAsAtomicUnit=on
  v2M_4 : MATLAB Function  TreatAsAtomicUnit=on
  v2M_5 : MATLAB Function  TreatAsAtomicUnit=on
  J_v_5(q) : Outport
  wires:
  R_1^0/1 -> J_v_1/1(R)
  J_v_1/1(J_v) -> v2M_1/1(v1)
  v2M_1/1(M) -> v2M_2/1(v1)
  v2M_2/1(M) -> v2M_3/1(v1)
  v2M_3/1(M) -> v2M_4/1(v1)
  v2M_4/1(M) -> v2M_5/1(v1)
  v2M_5/1(M) -> J_v_5(q)/1
  J_v_2/1(J_v) -> v2M_1/2(v2)
  J_v_3/1(J_v) -> v2M_2/2(v2)
  J_v_4/1(J_v) -> v2M_3/2(v2)
  Constant/1 -> v2M_4/2(v2), v2M_5/2(v2)
  R_2^0/1 -> J_v_2/1(R)
  R_3^0/1 -> J_v_3/1(R)
  R_4^0/1 -> J_v_4/1(R)
  p_1^0/1 -> J_v_1/2(p)
  p_2^0/1 -> J_v_2/2(p)
  p_3^0/1 -> J_v_3/2(p)
  p_4^0/1 -> J_v_4/2(p)
  type2/1 -> J_v_2/4(type)
  type1/1 -> J_v_1/4(type)
  type3/1 -> J_v_3/4(type)
  type4/1 -> J_v_4/4(type)
  p_5^0/1 -> J_v_1/3(pn), J_v_2/3(pn), J_v_3/3(pn), J_v_4/3(pn)

== system Dynamics/DYNAMIC/Jacobian/J_v/J_v_1 ==
  R : Inport
  p : Inport  Port=2
  pn : Inport  Port=3
  type : Inport  Port=4
  Add : Sum
  If : If  IfExpression=u1 == 1
  Prismatic Action : Subsystem  TreatAsAtomicUnit=on
  Revolute Action : Subsystem  TreatAsAtomicUnit=on
  J_v : Outport
  wires:
  type/1 -> If/1
  If/1 -> Revolute Action/Action
  If/2 -> Prismatic Action/Action
  Revolute Action/1(J_v) -> Add/1
  Prismatic Action/1(J_v) -> Add/2
  Add/1 -> J_v/1
  R/1 -> Prismatic Action/1(R), Revolute Action/1(R)
  p/1 -> Revolute Action/2(p)
  pn/1 -> Revolute Action/3(pn)

== system Dynamics/DYNAMIC/Jacobian/J_v/J_v_2 ==
  R : Inport
  p : Inport  Port=2
  pn : Inport  Port=3
  type : Inport  Port=4
  Add : Sum
  If : If  IfExpression=u1 == 1
  Prismatic Action : Subsystem  TreatAsAtomicUnit=on
  Revolute Action : Subsystem  TreatAsAtomicUnit=on
  J_v : Outport
  wires:
  type/1 -> If/1
  If/1 -> Revolute Action/Action
  If/2 -> Prismatic Action/Action
  Revolute Action/1(J_v) -> Add/1
  Prismatic Action/1(J_v) -> Add/2
  Add/1 -> J_v/1
  R/1 -> Prismatic Action/1(R), Revolute Action/1(R)
  p/1 -> Revolute Action/2(p)
  pn/1 -> Revolute Action/3(pn)

== system Dynamics/DYNAMIC/Jacobian/J_v/J_v_3 ==
  R : Inport
  p : Inport  Port=2
  pn : Inport  Port=3
  type : Inport  Port=4
  Add : Sum
  If : If  IfExpression=u1 == 1
  Prismatic Action : Subsystem  TreatAsAtomicUnit=on
  Revolute Action : Subsystem  TreatAsAtomicUnit=on
  J_v : Outport
  wires:
  type/1 -> If/1
  If/1 -> Revolute Action/Action
  If/2 -> Prismatic Action/Action
  Revolute Action/1(J_v) -> Add/1
  Prismatic Action/1(J_v) -> Add/2
  Add/1 -> J_v/1
  R/1 -> Prismatic Action/1(R), Revolute Action/1(R)
  p/1 -> Revolute Action/2(p)
  pn/1 -> Revolute Action/3(pn)

== system Dynamics/DYNAMIC/Jacobian/J_v/J_v_4 ==
  R : Inport
  p : Inport  Port=2
  pn : Inport  Port=3
  type : Inport  Port=4
  Add : Sum
  If : If  IfExpression=u1 == 1
  Prismatic Action : Subsystem  TreatAsAtomicUnit=on
  Revolute Action : Subsystem  TreatAsAtomicUnit=on
  J_v : Outport
  wires:
  type/1 -> If/1
  If/1 -> Revolute Action/Action
  If/2 -> Prismatic Action/Action
  Revolute Action/1(J_v) -> Add/1
  Prismatic Action/1(J_v) -> Add/2
  Add/1 -> J_v/1
  R/1 -> Prismatic Action/1(R), Revolute Action/1(R)
  p/1 -> Revolute Action/2(p)
  pn/1 -> Revolute Action/3(pn)

== system Dynamics/DYNAMIC/Jacobian/J_v/J_v_5 ==
  R : Inport
  p : Inport  Port=2
  pn : Inport  Port=3
  type : Inport  Port=4
  Add : Sum
  If : If  IfExpression=u1 == 1
  Prismatic Action : Subsystem  TreatAsAtomicUnit=on
  Revolute Action : Subsystem  TreatAsAtomicUnit=on
  J_v : Outport
  wires:
  type/1 -> If/1
  If/1 -> Revolute Action/Action
  If/2 -> Prismatic Action/Action
  Revolute Action/1(J_v) -> Add/1
  Prismatic Action/1(J_v) -> Add/2
  Add/1 -> J_v/1
  R/1 -> Prismatic Action/1(R), Revolute Action/1(R)
  p/1 -> Revolute Action/2(p)
  pn/1 -> Revolute Action/3(pn)

== system Dynamics/DYNAMIC/Jacobian/J_v/J_v_6 ==
  R : Inport
  p : Inport  Port=2
  pn : Inport  Port=3
  type : Inport  Port=4
  Add : Sum
  If : If  IfExpression=u1 == 1
  Prismatic Action : Subsystem  TreatAsAtomicUnit=on
  Revolute Action : Subsystem  TreatAsAtomicUnit=on
  J_v : Outport
  wires:
  type/1 -> If/1
  If/1 -> Revolute Action/Action
  If/2 -> Prismatic Action/Action
  Revolute Action/1(J_v) -> Add/1
  Prismatic Action/1(J_v) -> Add/2
  Add/1 -> J_v/1
  R/1 -> Prismatic Action/1(R), Revolute Action/1(R)
  p/1 -> Revolute Action/2(p)
  pn/1 -> Revolute Action/3(pn)

== system Dynamics/Subsystem/Jacobian/J(q) gen./J_v_1(q) ==
  Constant : Constant  Value=zeros(3,1)
  v2M_1 : MATLAB Function  TreatAsAtomicUnit=on
  v2M_2 : MATLAB Function  TreatAsAtomicUnit=on
  v2M_3 : MATLAB Function  TreatAsAtomicUnit=on
  v2M_4 : MATLAB Function  TreatAsAtomicUnit=on
  v2M_5 : MATLAB Function  TreatAsAtomicUnit=on
  J_v_1(q) : Outport
  wires:
  Constant/1 -> v2M_1/1(v1), v2M_5/2(v2), v2M_4/2(v2), v2M_3/2(v2), v2M_2/2(v2), v2M_1/2(v2)
  v2M_1/1(M) -> v2M_2/1(v1)
  v2M_2/1(M) -> v2M_3/1(v1)
  v2M_3/1(M) -> v2M_4/1(v1)
  v2M_4/1(M) -> v2M_5/1(v1)
  v2M_5/1(M) -> J_v_1(q)/1

== system Dynamics/Subsystem/Jacobian/J(q) gen./J_v_2(q) ==
  R_1^0 : Inport
  p_1^0 : Inport  Port=2
  p_2^0 : Inport  Port=3
  type1 : Inport  Port=4
  Constant : Constant  Value=zeros(3,1)
  J_v_1 : Subsystem
  v2M_1 : MATLAB Function  TreatAsAtomicUnit=on
  v2M_2 : MATLAB Function  TreatAsAtomicUnit=on
  v2M_3 : MATLAB Function  TreatAsAtomicUnit=on
  v2M_4 : MATLAB Function  TreatAsAtomicUnit=on
  v2M_5 : MATLAB Function  TreatAsAtomicUnit=on
  J_v_2(q) : Outport
  wires:
  R_1^0/1 -> J_v_1/1(R)
  J_v_1/1(J_v) -> v2M_1/1(v1)
  v2M_1/1(M) -> v2M_2/1(v1)
  v2M_2/1(M) -> v2M_3/1(v1)
  v2M_3/1(M) -> v2M_4/1(v1)
  v2M_4/1(M) -> v2M_5/1(v1)
  v2M_5/1(M) -> J_v_2(q)/1
  Constant/1 -> v2M_3/2(v2), v2M_4/2(v2), v2M_5/2(v2), v2M_1/2(v2), v2M_2/2(v2)
  p_1^0/1 -> J_v_1/2(p)
  type1/1 -> J_v_1/4(type)
  p_2^0/1 -> J_v_1/3(pn)

== system Dynamics/Subsystem/Jacobian/J(q) gen./J_v_3(q) ==
  R_1^0 : Inport
  R_2^0 : Inport  Port=2
  p_1^0 : Inport  Port=3
  p_2^0 : Inport  Port=4
  p_3^0 : Inport  Port=5
  type1 : Inport  Port=6
  type2 : Inport  Port=7
  Constant : Constant  Value=zeros(3,1)
  J_v_1 : Subsystem
  J_v_2 : Subsystem
  v2M_1 : MATLAB Function  TreatAsAtomicUnit=on
  v2M_2 : MATLAB Function  TreatAsAtomicUnit=on
  v2M_3 : MATLAB Function  TreatAsAtomicUnit=on
  v2M_4 : MATLAB Function  TreatAsAtomicUnit=on
  v2M_5 : MATLAB Function  TreatAsAtomicUnit=on
  J_v_3(q) : Outport
  wires:
  R_1^0/1 -> J_v_1/1(R)
  J_v_1/1(J_v) -> v2M_1/1(v1)
  v2M_1/1(M) -> v2M_2/1(v1)
  v2M_2/1(M) -> v2M_3/1(v1)
  v2M_3/1(M) -> v2M_4/1(v1)
  v2M_4/1(M) -> v2M_5/1(v1)
  v2M_5/1(M) -> J_v_3(q)/1
  J_v_2/1(J_v) -> v2M_1/2(v2)
  Constant/1 -> v2M_5/2(v2), v2M_4/2(v2), v2M_2/2(v2), v2M_3/2(v2)
  R_2^0/1 -> J_v_2/1(R)
  p_1^0/1 -> J_v_1/2(p)
  p_2^0/1 -> J_v_2/2(p)
  type2/1 -> J_v_2/4(type)
  type1/1 -> J_v_1/4(type)
  p_3^0/1 -> J_v_1/3(pn), J_v_2/3(pn)

== system Dynamics/Subsystem/Jacobian/J(q) gen./J_v_4(q) ==
  R_1^0 : Inport
  R_2^0 : Inport  Port=2
  R_3^0 : Inport  Port=3
  p_1^0 : Inport  Port=4
  p_2^0 : Inport  Port=5
  p_3^0 : Inport  Port=6
  p_4^0 : Inport  Port=7
  type1 : Inport  Port=8
  type2 : Inport  Port=9
  type3 : Inport  Port=10
  Constant : Constant  Value=zeros(3,1)
  J_v_1 : Subsystem
  J_v_2 : Subsystem
  J_v_3 : Subsystem
  v2M_1 : MATLAB Function  TreatAsAtomicUnit=on
  v2M_2 : MATLAB Function  TreatAsAtomicUnit=on
  v2M_3 : MATLAB Function  TreatAsAtomicUnit=on
  v2M_4 : MATLAB Function  TreatAsAtomicUnit=on
  v2M_5 : MATLAB Function  TreatAsAtomicUnit=on
  J_v_4(q) : Outport
  wires:
  R_1^0/1 -> J_v_1/1(R)
  J_v_1/1(J_v) -> v2M_1/1(v1)
  v2M_1/1(M) -> v2M_2/1(v1)
  v2M_2/1(M) -> v2M_3/1(v1)
  v2M_3/1(M) -> v2M_4/1(v1)
  v2M_4/1(M) -> v2M_5/1(v1)
  v2M_5/1(M) -> J_v_4(q)/1
  J_v_2/1(J_v) -> v2M_1/2(v2)
  J_v_3/1(J_v) -> v2M_2/2(v2)
  Constant/1 -> v2M_5/2(v2), v2M_3/2(v2), v2M_4/2(v2)
  R_2^0/1 -> J_v_2/1(R)
  R_3^0/1 -> J_v_3/1(R)
  p_1^0/1 -> J_v_1/2(p)
  p_2^0/1 -> J_v_2/2(p)
  p_3^0/1 -> J_v_3/2(p)
  type2/1 -> J_v_2/4(type)
  type1/1 -> J_v_1/4(type)
  type3/1 -> J_v_3/4(type)
  p_4^0/1 -> J_v_1/3(pn), J_v_2/3(pn), J_v_3/3(pn)

== system Dynamics/Subsystem/Jacobian/J(q) gen./J_v_5(q) ==
  R_1^0 : Inport
  R_2^0 : Inport  Port=2
  R_3^0 : Inport  Port=3
  R_4^0 : Inport  Port=4
  p_1^0 : Inport  Port=5
  p_2^0 : Inport  Port=6
  p_3^0 : Inport  Port=7
  p_4^0 : Inport  Port=8
  p_5^0 : Inport  Port=9
  type1 : Inport  Port=10
  type2 : Inport  Port=11
  type3 : Inport  Port=12
  type4 : Inport  Port=13
  Constant : Constant  Value=zeros(3,1)
  J_v_1 : Subsystem
  J_v_2 : Subsystem
  J_v_3 : Subsystem
  J_v_4 : Subsystem
  v2M_1 : MATLAB Function  TreatAsAtomicUnit=on
  v2M_2 : MATLAB Function  TreatAsAtomicUnit=on
  v2M_3 : MATLAB Function  TreatAsAtomicUnit=on
  v2M_4 : MATLAB Function  TreatAsAtomicUnit=on
  v2M_5 : MATLAB Function  TreatAsAtomicUnit=on
  J_v_5(q) : Outport
  wires:
  R_1^0/1 -> J_v_1/1(R)
  J_v_1/1(J_v) -> v2M_1/1(v1)
  v2M_1/1(M) -> v2M_2/1(v1)
  v2M_2/1(M) -> v2M_3/1(v1)
  v2M_3/1(M) -> v2M_4/1(v1)
  v2M_4/1(M) -> v2M_5/1(v1)
  v2M_5/1(M) -> J_v_5(q)/1
  J_v_2/1(J_v) -> v2M_1/2(v2)
  J_v_3/1(J_v) -> v2M_2/2(v2)
  J_v_4/1(J_v) -> v2M_3/2(v2)
  Constant/1 -> v2M_4/2(v2), v2M_5/2(v2)
  R_2^0/1 -> J_v_2/1(R)
  R_3^0/1 -> J_v_3/1(R)
  R_4^0/1 -> J_v_4/1(R)
  p_1^0/1 -> J_v_1/2(p)
  p_2^0/1 -> J_v_2/2(p)
  p_3^0/1 -> J_v_3/2(p)
  p_4^0/1 -> J_v_4/2(p)
  type2/1 -> J_v_2/4(type)
  type1/1 -> J_v_1/4(type)
  type3/1 -> J_v_3/4(type)
  type4/1 -> J_v_4/4(type)
  p_5^0/1 -> J_v_1/3(pn), J_v_2/3(pn), J_v_3/3(pn), J_v_4/3(pn)

== system Dynamics/Subsystem/Jacobian/J_v/J_v_1 ==
  R : Inport
  p : Inport  Port=2
  pn : Inport  Port=3
  type : Inport  Port=4
  Add : Sum
  If : If  IfExpression=u1 == 1
  Prismatic Action : Subsystem  TreatAsAtomicUnit=on
  Revolute Action : Subsystem  TreatAsAtomicUnit=on
  J_v : Outport
  wires:
  type/1 -> If/1
  If/1 -> Revolute Action/Action
  If/2 -> Prismatic Action/Action
  Revolute Action/1(J_v) -> Add/1
  Prismatic Action/1(J_v) -> Add/2
  Add/1 -> J_v/1
  R/1 -> Prismatic Action/1(R), Revolute Action/1(R)
  p/1 -> Revolute Action/2(p)
  pn/1 -> Revolute Action/3(pn)

== system Dynamics/Subsystem/Jacobian/J_v/J_v_2 ==
  R : Inport
  p : Inport  Port=2
  pn : Inport  Port=3
  type : Inport  Port=4
  Add : Sum
  If : If  IfExpression=u1 == 1
  Prismatic Action : Subsystem  TreatAsAtomicUnit=on
  Revolute Action : Subsystem  TreatAsAtomicUnit=on
  J_v : Outport
  wires:
  type/1 -> If/1
  If/1 -> Revolute Action/Action
  If/2 -> Prismatic Action/Action
  Revolute Action/1(J_v) -> Add/1
  Prismatic Action/1(J_v) -> Add/2
  Add/1 -> J_v/1
  R/1 -> Prismatic Action/1(R), Revolute Action/1(R)
  p/1 -> Revolute Action/2(p)
  pn/1 -> Revolute Action/3(pn)

== system Dynamics/Subsystem/Jacobian/J_v/J_v_3 ==
  R : Inport
  p : Inport  Port=2
  pn : Inport  Port=3
  type : Inport  Port=4
  Add : Sum
  If : If  IfExpression=u1 == 1
  Prismatic Action : Subsystem  TreatAsAtomicUnit=on
  Revolute Action : Subsystem  TreatAsAtomicUnit=on
  J_v : Outport
  wires:
  type/1 -> If/1
  If/1 -> Revolute Action/Action
  If/2 -> Prismatic Action/Action
  Revolute Action/1(J_v) -> Add/1
  Prismatic Action/1(J_v) -> Add/2
  Add/1 -> J_v/1
  R/1 -> Prismatic Action/1(R), Revolute Action/1(R)
  p/1 -> Revolute Action/2(p)
  pn/1 -> Revolute Action/3(pn)

== system Dynamics/Subsystem/Jacobian/J_v/J_v_4 ==
  R : Inport
  p : Inport  Port=2
  pn : Inport  Port=3
  type : Inport  Port=4
  Add : Sum
  If : If  IfExpression=u1 == 1
  Prismatic Action : Subsystem  TreatAsAtomicUnit=on
  Revolute Action : Subsystem  TreatAsAtomicUnit=on
  J_v : Outport
  wires:
  type/1 -> If/1
  If/1 -> Revolute Action/Action
  If/2 -> Prismatic Action/Action
  Revolute Action/1(J_v) -> Add/1
  Prismatic Action/1(J_v) -> Add/2
  Add/1 -> J_v/1
  R/1 -> Prismatic Action/1(R), Revolute Action/1(R)
  p/1 -> Revolute Action/2(p)
  pn/1 -> Revolute Action/3(pn)

== system Dynamics/Subsystem/Jacobian/J_v/J_v_5 ==
  R : Inport
  p : Inport  Port=2
  pn : Inport  Port=3
  type : Inport  Port=4
  Add : Sum
  If : If  IfExpression=u1 == 1
  Prismatic Action : Subsystem  TreatAsAtomicUnit=on
  Revolute Action : Subsystem  TreatAsAtomicUnit=on
  J_v : Outport
  wires:
  type/1 -> If/1
  If/1 -> Revolute Action/Action
  If/2 -> Prismatic Action/Action
  Revolute Action/1(J_v) -> Add/1
  Prismatic Action/1(J_v) -> Add/2
  Add/1 -> J_v/1
  R/1 -> Prismatic Action/1(R), Revolute Action/1(R)
  p/1 -> Revolute Action/2(p)
  pn/1 -> Revolute Action/3(pn)

== system Dynamics/Subsystem/Jacobian/J_v/J_v_6 ==
  R : Inport
  p : Inport  Port=2
  pn : Inport  Port=3
  type : Inport  Port=4
  Add : Sum
  If : If  IfExpression=u1 == 1
  Prismatic Action : Subsystem  TreatAsAtomicUnit=on
  Revolute Action : Subsystem  TreatAsAtomicUnit=on
  J_v : Outport
  wires:
  type/1 -> If/1
  If/1 -> Revolute Action/Action
  If/2 -> Prismatic Action/Action
  Revolute Action/1(J_v) -> Add/1
  Prismatic Action/1(J_v) -> Add/2
  Add/1 -> J_v/1
  R/1 -> Prismatic Action/1(R), Revolute Action/1(R)
  p/1 -> Revolute Action/2(p)
  pn/1 -> Revolute Action/3(pn)

== system Dynamics/Subsystem2/Jacobian/J(q) gen./J_v_1(q) ==
  Constant : Constant  Value=zeros(3,1)
  v2M_1 : MATLAB Function  TreatAsAtomicUnit=on
  v2M_2 : MATLAB Function  TreatAsAtomicUnit=on
  v2M_3 : MATLAB Function  TreatAsAtomicUnit=on
  v2M_4 : MATLAB Function  TreatAsAtomicUnit=on
  v2M_5 : MATLAB Function  TreatAsAtomicUnit=on
  J_v_1(q) : Outport
  wires:
  Constant/1 -> v2M_1/1(v1), v2M_5/2(v2), v2M_4/2(v2), v2M_3/2(v2), v2M_2/2(v2), v2M_1/2(v2)
  v2M_1/1(M) -> v2M_2/1(v1)
  v2M_2/1(M) -> v2M_3/1(v1)
  v2M_3/1(M) -> v2M_4/1(v1)
  v2M_4/1(M) -> v2M_5/1(v1)
  v2M_5/1(M) -> J_v_1(q)/1
